simulink model "motor_realista"  (R2020b)
settings: Solver=VariableStepAuto  StartTime=0.0  StopTime=10.0  MaxStep=1e-5  RelTol=1e-3
values from neighbouring files (symbols this model uses):
  T = u    [pendulo_estimador.m]
undefined symbols (not defined in the file or in its folder): pos_ini
libraries: simulink x3
settings Model: Creator=abierto  LastModifiedBy=noether
settings SFSimCC: CustomCodeUndefinedFunction=UseInterfaceOnly

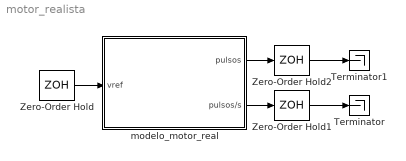
== system motor_realista ==
  Terminator : Terminator
  Terminator1 : Terminator
  Zero-Order Hold : ZeroOrderHold  SampleTime=T
  Zero-Order Hold1 : ZeroOrderHold  SampleTime=T
  Zero-Order Hold2 : ZeroOrderHold  SampleTime=T
  modelo_motor_real : Subsystem
  wires:
  Zero-Order Hold/1 -> modelo_motor_real/1(vref)
  modelo_motor_real/1(pulsos) -> Zero-Order Hold2/1
  Zero-Order Hold2/1 -> Terminator1/1
  modelo_motor_real/2(pulsos/s) -> Zero-Order Hold1/1
  Zero-Order Hold1/1 -> Terminator/1

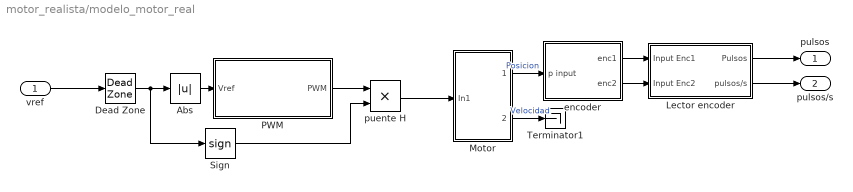
== system motor_realista/modelo_motor_real ==
  vref : Inport
  Abs : Abs
  Dead Zone : DeadZone  SaturateOnIntegerOverflow=on
  Lector encoder : Subsystem
  Motor : Subsystem  mask{Ke=100, P=50}
  PWM : Subsystem  mask{T=0.0001, Vmax=12}
      mask prompts: T "Periodo"; Vmax "Voltaje Fuente"
  Sign : Signum
  Terminator1 : Terminator
  encoder : Subsystem
  puente H : Product
  pulsos : Outport  VectorParamsAs1DForOutWhenUnconnected=off
  pulsos/s : Outport  Port=2  VectorParamsAs1DForOutWhenUnconnected=off
  wires:
  Motor/1(p. (rad)) -> encoder/1(p input)  "Posicion"
  Abs/1 -> PWM/1(Vref)
  Motor/2(v. (rad/s)) -> Terminator1/1  "Velocidad"
  PWM/1(PWM) -> puente H/1
  Sign/1 -> puente H/2
  Dead Zone/1 -> Sign/1, Abs/1
  encoder/1(enc1) -> Lector encoder/1(Input Enc1)
  encoder/2(enc2) -> Lector encoder/2(Input Enc2)
  vref/1 -> Dead Zone/1
  Lector encoder/2(pulsos/s) -> pulsos/s/1
  Lector encoder/1(Pulsos) -> pulsos/1
  puente H/1 -> Motor/1(In1)

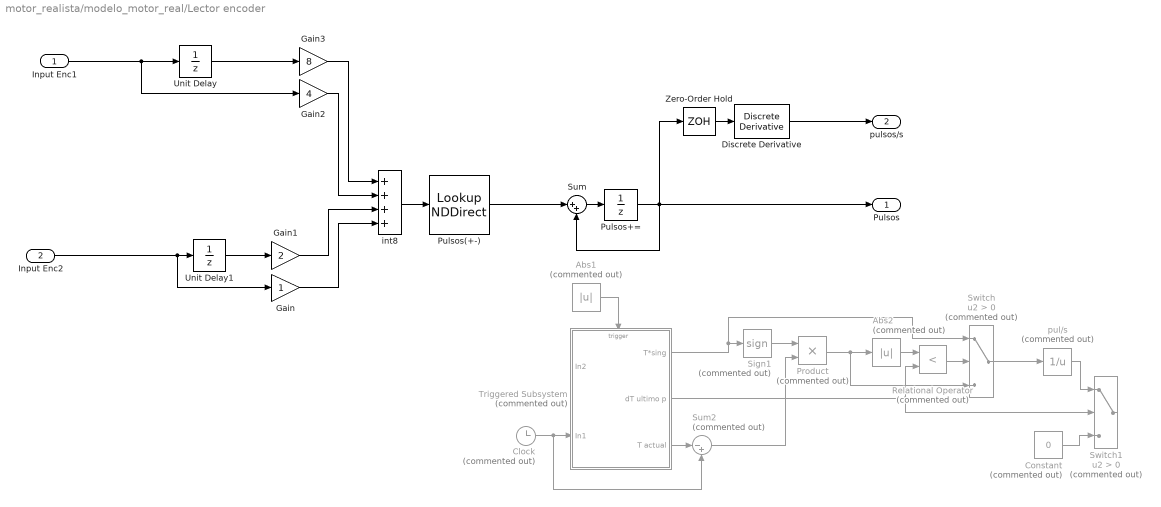
== system motor_realista/modelo_motor_real/Lector encoder ==
  Input Enc1 : Inport
  Input Enc2 : Inport  Port=2
  Abs1 : Abs  Commented=on
  Abs2 : Abs  Commented=on
  Clock : Clock  Commented=on
      settings: Decimation=100
  Constant : Constant  Commented=on  Value=0
  Discrete Derivative : simulink/Discrete/Discrete Derivative  gainval=1.0  ICPrevScaledInput=0.0  OutMin=[]  OutMax=[]  OutDataType=fixdt(1, 16)  OutScaling=2^-10  DoSatur=off
  Gain : Gain
  Gain1 : Gain  Gain=2
  Gain2 : Gain  Gain=4
  Gain3 : Gain  Gain=8
  Product : Product  Commented=on
  Pulsos(+-) : LookupNDDirect  NumberOfTableDimensions=1  Table=[0 -1 1 0 1 10 10 -1 -1 10 10 1 0 1 -1 0];
  Pulsos+= : UnitDelay  InitialCondition=pos_ini  SampleTime=-1  HasFrameUpgradeWarning=on
  Relational Operator : RelationalOperator  Commented=on  Operator=<  OutDataTypeStr=boolean  RndMeth=Simplest
  Sign1 : Signum  Commented=on
  Sum : Sum  Inputs=|++
  Sum2 : Sum  Commented=on  Inputs=|-+
  Switch : Switch  Commented=on  Criteria=u2 > Threshold
  Switch1 : Switch  Commented=on  Criteria=u2 > Threshold
  Triggered Subsystem : Subsystem  Commented=on  TreatAsAtomicUnit=on
  Unit Delay : UnitDelay  SampleTime=0.0001  HasFrameUpgradeWarning=on
  Unit Delay1 : UnitDelay  SampleTime=0.0001  HasFrameUpgradeWarning=on
  Zero-Order Hold : ZeroOrderHold
  int8 : Sum  Inputs=++++
  pul/s : Math  Commented=on  Operator=reciprocal  SignedPower=on  SaturateOnIntegerOverflow=on
  Pulsos : Outport  VectorParamsAs1DForOutWhenUnconnected=off
  pulsos/s : Outport  Port=2  VectorParamsAs1DForOutWhenUnconnected=off
  wires:
  int8/1 -> Pulsos(+-)/1
  Gain/1 -> int8/4
  Gain3/1 -> int8/1
  Sum/1 -> Pulsos+=/1
  Unit Delay1/1 -> Gain1/1
  Unit Delay/1 -> Gain3/1
  Input Enc2/1 -> Gain/1, Unit Delay1/1
  Gain2/1 -> int8/2
  Pulsos(+-)/1 -> Sum/1
  Gain1/1 -> int8/3
  Input Enc1/1 -> Unit Delay/1, Gain2/1
  Pulsos+=/1 -> Zero-Order Hold/1, Pulsos/1, Sum/2
  Clock/1 -> Triggered Subsystem/2(In1), Sum2/2
  Switch/1 -> pul/s/1
  Triggered Subsystem/1("T*sing ") -> Sign1/1, Switch/1
  Triggered Subsystem/3(T actual) -> Sum2/1
  Abs1/1 -> Triggered Subsystem/Trigger
  Triggered Subsystem/2("dT ultimo p ") -> Switch1/2, Relational Operator/2
  Abs2/1 -> Relational Operator/1
  Relational Operator/1 -> Switch/2
  Product/1 -> Switch/3, Abs2/1
  Sign1/1 -> Product/1
  Sum2/1 -> Product/2
  pul/s/1 -> Switch1/1
  Constant/1 -> Switch1/3
  Zero-Order Hold/1 -> Discrete Derivative/1
  Discrete Derivative/1 -> pulsos/s/1

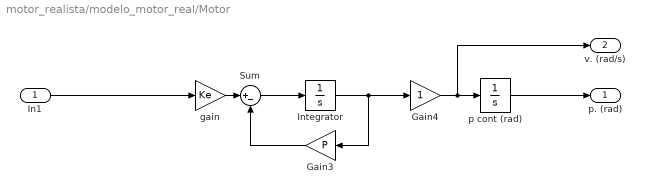
== system motor_realista/modelo_motor_real/Motor ==
  In1 : Inport
  Gain3 : Gain  Gain=P
  Gain4 : Gain
  Integrator : Integrator
  Sum : Sum  Inputs=|+-
  gain : Gain  Gain=Ke
  p cont (rad) : Integrator  InitialCondition=pos_ini
  p. (rad) : Outport  VectorParamsAs1DForOutWhenUnconnected=off
  v. (rad/s) : Outport  Port=2  VectorParamsAs1DForOutWhenUnconnected=off
  wires:
  p cont (rad)/1 -> p. (rad)/1
  Gain3/1 -> Sum/2
  Gain4/1 -> v. (rad/s)/1, p cont (rad)/1
  Sum/1 -> Integrator/1
  gain/1 -> Sum/1
  Integrator/1 -> Gain4/1, Gain3/1
  In1/1 -> gain/1

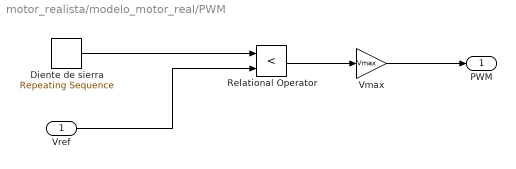
== system motor_realista/modelo_motor_real/PWM ==
  Vref : Inport
  Diente de sierra : simulink/Sources/Repeating Sequence  rep_seq_t=linspace(0,T,100)  rep_seq_y=linspace(0,Vmax,100)
  Relational Operator : RelationalOperator  Operator=<  OutDataTypeStr=boolean  RndMeth=Simplest
  Vmax : Gain  Gain=Vmax
  PWM : Outport  VectorParamsAs1DForOutWhenUnconnected=off
  wires:
  Diente de sierra/1 -> Relational Operator/1
  Relational Operator/1 -> Vmax/1
  Vmax/1 -> PWM/1
  Vref/1 -> Relational Operator/2

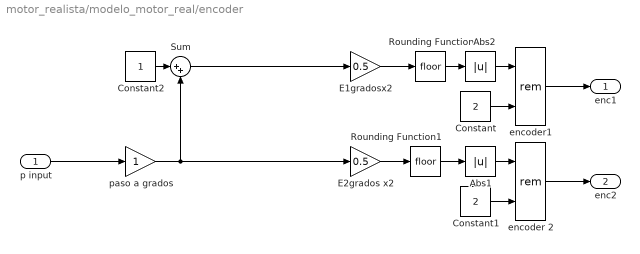
== system motor_realista/modelo_motor_real/encoder ==
  p input : Inport
  Abs1 : Abs
  Abs2 : Abs
  Constant : Constant  Value=2
  Constant1 : Constant  Value=2
  Constant2 : Constant
  E1gradosx2 : Gain  Gain=0.5
  E2grados x2 : Gain  Gain=0.5
  Rounding Function : Rounding
  Rounding Function1 : Rounding
  Sum : Sum  Inputs=|++
  encoder 2 : Math  Operator=rem  SignedPower=on  SaturateOnIntegerOverflow=on
  encoder1 : Math  Operator=rem  SignedPower=on  SaturateOnIntegerOverflow=on
  paso a grados : Gain
  enc1 : Outport  VectorParamsAs1DForOutWhenUnconnected=off
  enc2 : Outport  Port=2  VectorParamsAs1DForOutWhenUnconnected=off
  wires:
  p input/1 -> paso a grados/1
  encoder 2/1 -> enc2/1
  encoder1/1 -> enc1/1
  Constant1/1 -> encoder 2/2
  Constant/1 -> encoder1/2
  Rounding Function1/1 -> Abs1/1
  E2grados x2/1 -> Rounding Function1/1
  paso a grados/1 -> E2grados x2/1, Sum/2
  E1gradosx2/1 -> Rounding Function/1
  Constant2/1 -> Sum/1
  Sum/1 -> E1gradosx2/1
  Abs2/1 -> encoder1/1
  Rounding Function/1 -> Abs2/1
  Abs1/1 -> encoder 2/1

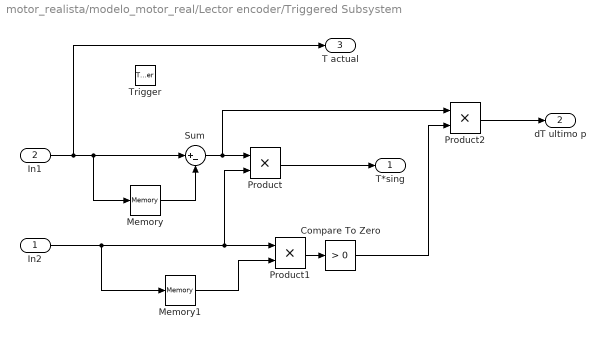
== system motor_realista/modelo_motor_real/Lector encoder/Triggered Subsystem ==
  In2 : Inport
  In1 : Inport  Port=2
  Trigger : TriggerPort  VariantControl=Variant
  Compare To Zero : simulink/Logic and Bit Operations/Compare To Zero  relop=>  OutDataTypeStr=boolean
  Memory : Memory  InheritSampleTime=on
  Memory1 : Memory  InheritSampleTime=on
  Product : Product
  Product1 : Product
  Product2 : Product
  Sum : Sum  Inputs=|+-
  "T*sing " : Outport  VectorParamsAs1DForOutWhenUnconnected=off
  "dT ultimo p " : Outport  Port=2  VectorParamsAs1DForOutWhenUnconnected=off
  T actual : Outport  Port=3  VectorParamsAs1DForOutWhenUnconnected=off
  wires:
  Memory/1 -> Sum/2
  Sum/1 -> Product2/1, Product/1
  Product/1 -> "T*sing "/1
  In2/1 -> Memory1/1, Product/2, Product1/1
  In1/1 -> T actual/1, Sum/1, Memory/1
  Memory1/1 -> Product1/2
  Product1/1 -> Compare To Zero/1
  Product2/1 -> "dT ultimo p "/1
  Compare To Zero/1 -> Product2/2
